simulink model "PowerTransmissionModel"  (R2024b)
settings: Solver=VariableStepAuto  StartTime=0.0  StopTime=1  RelTol=1e-3
libraries: fl_lib x17, ee_lib x10, nesl_utility x7
settings Model: Creator=pvenupra  LastModifiedBy=alial

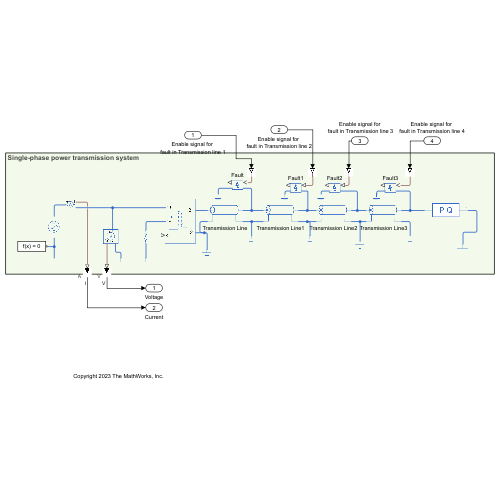
[thumbnail: Simulink's stored preview of the top-level diagram]
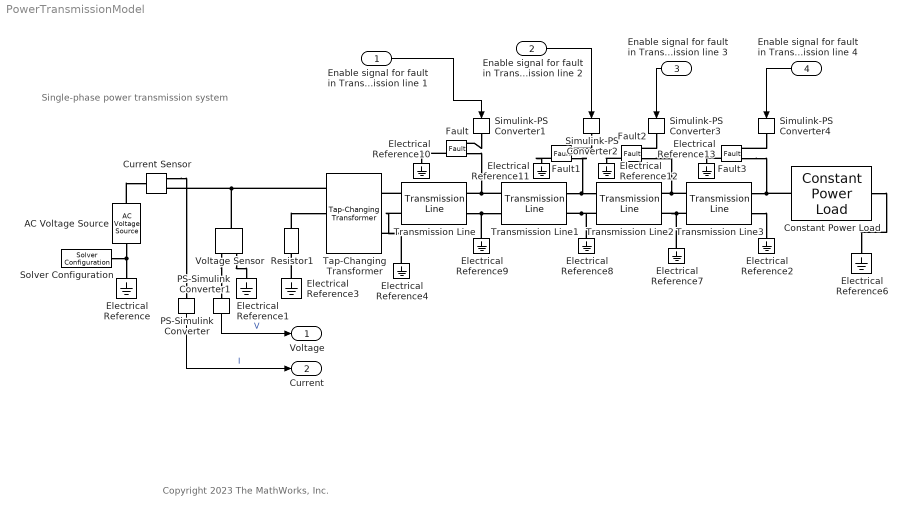
== system PowerTransmissionModel ==
  note: Copyright 2023 The MathWorks, Inc.
  note: Single-phase power transmission system
  Enable signal for fault in Transmission line 1 : Inport  SampleTime=0.025
  Enable signal for fault in Transmission line 2 : Inport  Port=2  SampleTime=0.025
  Enable signal for fault in Transmission line 3 : Inport  Port=3  SampleTime=0.025
  Enable signal for fault in Transmission line 4 : Inport  Port=4  SampleTime=0.025
  AC Voltage Source : fl_lib/Electrical/Electrical Sources/AC Voltage Source  amp=10 kV  shift=0 deg  frequency=60 Hz
  Constant Power Load : ee_lib/Passive/Constant Power Load  load_type=ee.enum.dc_ac.ac  consumed_power=100 W  min_supply_voltage=20 V  G_reverse=1e-6 S  deltaV=1e-3 V  active_power=4e5 W  reactive_power=1e5 A*V  f0=60 Hz  Vrms_min=400 V  tau=0.01 s  Vrms_ini=400 V  Vang_ini=0 deg  fault_action=simscape.enum.assert.action.none  t_fault=1 s
      settings: InternalSimscapePortConfiguration="{\"Bottom\":[],\"Left\":[{\"id\":\"p\",\"label\":\"+\",\"type\":\"foundation.electrical.electrical\"}],\"Right\":[{\"id\":\"n\",\"label\":\"-\",\"type\":\"foundation.electrical.electrical\"}],\"Top\":[]}"
  Current Sensor : fl_lib/Electrical/Electrical Sensors/Current Sensor
  Electrical Reference{,1..4,6..13} (13 alike) : fl_lib/Electrical/Electrical Elements/Electrical Reference
  Fault{,1..3} (4 alike) : ee_lib/Utilities/Fault  R_unfaulted=inf Ohm  R_faulted=1e-3 Ohm  fault_action=1  enable_temporal_fault=0  t_fault=0.3 s  fault_duration=inf s  enable_behavioral_fault=0  permissible_voltage_range=[-100, 100] V  t_fail_on_voltage=1 s  permissible_current_range=[-1, 1] A  t_fail_on_current=1 s  enable_external_fault=1  fault_condition=1  fault_threshold=0.5  fault_resettable=1
      settings: InternalSimscapePortConfiguration="{\"Bottom\":[],\"Left\":[{\"id\":\"p\",\"label\":\"+\",\"type\":\"foundation.electrical.electrical\"},{\"id\":\"F\",\"label\":\"F\",\"type\":\"input\"}],\"Right\":[{\"id\":\"n\",\"label\":\"-\",\"type\":\"foundation.electrical.electrical\"},{\"id\":\"X\",\"label\":\"X\",\"type\":\"output\"}],\"Top\":[]}"
  PS-Simulink Converter : nesl_utility/PS-Simulink Converter  PhysicalDomain=network_engine_domain  SubClassName=ps_output  LeftPortType=input  RightPortType=output  PseudoPeriodic=off  Frequencies=[]  VectorFormat=1-D array  Unit=A  AffineConversion=off
  PS-Simulink Converter1 : nesl_utility/PS-Simulink Converter  PhysicalDomain=network_engine_domain  SubClassName=ps_output  LeftPortType=input  RightPortType=output  PseudoPeriodic=off  Frequencies=[]  VectorFormat=1-D array  Unit=V  AffineConversion=off
  Resistor1 : fl_lib/Electrical/Electrical Elements/Resistor  R=0.2 Ohm  i_specify=off  i_priority=None  i=0 A  i_nominal_specify=off  i_nominal_value=1  i_nominal_unit=A  v_specify=off  v_priority=None  v=0 V  v_nominal_specify=off  v_nominal_value=1  v_nominal_unit=V
  Simulink-PS Converter{1..4} (4 alike) : nesl_utility/Simulink-PS Converter  PhysicalDomain=network_engine_domain  SubClassName=ps_input  LeftPortType=input  RightPortType=output  PseudoPeriodic=off  Frequencies=[]  NoiseDistribution=none  NoiseParameters=[]  Unit=1  AffineConversion=off  FilteringAndDerivatives=provide  SimscapeFilterOrder=1  InputFilterTimeConstant=0.001  UdotUserProvided=0
  Solver Configuration : nesl_utility/Solver Configuration  PhysicalDomain=network_engine_domain  SubClassName=solver  LeftPortType=input  RightPortType=generic  Tones=[]  Harmonics=[]  SimulateNoise=off  Profile=off  UseLocalSampling=off  EnableSwitchedLinearOptims=on  FrequencyDomain=off  UseCCode=off  RelTol=0.001  AbsTol=1e-06  MinStep=1e-09  ToWorkspace=off  RevertToSquareIcSolve=off  NumHomotopyIterations=100  PhasorMode=off  PhasorModeNumHarmonics=1  ConsistencySolver=NEWTON_FTOL  IndexReductionMethod=DerivativeReplacement  DoDC=off  ResidualTolerance=1e-09  ConsistencyTolSource=GLOBAL  ConsistencyAbsTol=0.001  ConsistencyRelTol=0.001  ConsistencyTolFactor=0.001  UseLocalSolver=on  LocalSolverChoice=NE_BACKWARD_EULER_ADVANCER  ResolveIndetEquations=on  FunctionEvalNumThread=1  LocalSolverSampleTime=1e-4  DoFixedCost=on  MaxNonlinIter=3  MaxModeIter=2  ComputeImpulses=off  ImpulseIterations=2  LinearAlgebra=auto  LinearAlgebraNumThread=0  EquationFormulation=NE_TIME_EF  DelaysMemoryBudget=1024  AutomaticFiltering=on  FilteringTimeConstant=0.001  PartitionStorageMethod=AS_NEEDED  PartitionMemoryBudget=1024  PartitionMethod=FAST  MultibodyUseLocalSolver=off  MultibodyLocalSolverChoice=ODE1  MultibodyLocalSolverSampleTime=0.001
  Tap-Changing Transformer : ee_lib/Passive/Transformers/Tap-Changing Transformer  n0=25  Lp=0.0133 H  Ls=2.12e-6 H  Rm=50 kOhm  Lm=132.63 H  Rp=2 Ohm  Rs="0.032  Ohm"  Gp=0 1/Ohm  Gs=0 1/Ohm  prm=1  pmin=-5  pmax=5  delta=1  controlThreshold=0.5  i1_specify=off  i1_priority=None  i1=0 A  i1_nominal_specify=off  i1_nominal_value=1  i1_nominal_unit=A  i2_specify=off  i2_priority=None  i2=0 A  i2_nominal_specify=off  i2_nominal_value=1  i2_nominal_unit=A  tapPosition_specify=off  tapPosition_priority=High  tapPosition=0
      settings: InternalSimscapePortConfiguration="{\"Bottom\":[],\"Left\":[{\"id\":\"p1\",\"label\":\"1+\",\"type\":\"foundation.electrical.electrical\"},{\"id\":\"n1\",\"label\":\"1-\",\"type\":\"foundation.electrical.electrical\"},{\"id\":\"control\",\"label\":\"c\",\"type\":\"input\"}],\"Right\":[{\"id\":\"p2\",\"label\":\"2+\",\"type\":\"foundation.electrical.electrical\"},{\"id\":\"n2\",\"label\":\"2-\",\"type\":\"foundation.electrical.electrical\"}],\"Top\":[]}"
  Transmission Line : ee_lib/Passive/Lines/Transmission Line  model_type=4  TD=5 ns  LC_param=2  Z0_delay_based=50 Ohm  Z0=50 Ohm  freq=60 Hz  Ll=220 uH/m  L=0.5 mH/km  C=0.3 uF/km  R=.2 Ohm/km  G=5e-6 S/m  LEN=0.1 km  N=1
      settings: InternalSimscapePortConfiguration="{\"Bottom\":[],\"Left\":[{\"id\":\"p1\",\"label\":\"\",\"type\":\"foundation.electrical.electrical\"},{\"id\":\"n1\",\"label\":\"\",\"type\":\"foundation.electrical.electrical\"}],\"Right\":[{\"id\":\"p2\",\"label\":\"\",\"type\":\"foundation.electrical.electrical\"},{\"id\":\"n2\",\"label\":\"\",\"type\":\"foundation.electrical.electrical\"}],\"Top\":[]}"
  Transmission Line1 : ee_lib/Passive/Lines/Transmission Line  model_type=4  TD=5 ns  LC_param=2  Z0_delay_based=50 Ohm  Z0=50 Ohm  freq=60 Hz  Ll=220 uH/m  L=0.5 mH/km  C=0.3 uF/km  R=.2 Ohm/km  G=5e-6 S/m  LEN=0.1 km  N=1
      settings: InternalSimscapePortConfiguration="{\"Bottom\":[],\"Left\":[{\"id\":\"p1\",\"label\":\"\",\"type\":\"foundation.electrical.electrical\"},{\"id\":\"n1\",\"label\":\"\",\"type\":\"foundation.electrical.electrical\"}],\"Right\":[{\"id\":\"p2\",\"label\":\"\",\"type\":\"foundation.electrical.electrical\"},{\"id\":\"n2\",\"label\":\"\",\"type\":\"foundation.electrical.electrical\"}],\"Top\":[]}"
  Transmission Line2 : ee_lib/Passive/Lines/Transmission Line  model_type=4  TD=5 ns  LC_param=2  Z0_delay_based=50 Ohm  Z0=50 Ohm  freq=60 Hz  Ll=220 uH/m  L=0.5 mH/km  C=0.3 uF/km  R=.2 Ohm/km  G=5e-6 S/m  LEN=0.1 km  N=1
      settings: InternalSimscapePortConfiguration="{\"Bottom\":[],\"Left\":[{\"id\":\"p1\",\"label\":\"\",\"type\":\"foundation.electrical.electrical\"},{\"id\":\"n1\",\"label\":\"\",\"type\":\"foundation.electrical.electrical\"}],\"Right\":[{\"id\":\"p2\",\"label\":\"\",\"type\":\"foundation.electrical.electrical\"},{\"id\":\"n2\",\"label\":\"\",\"type\":\"foundation.electrical.electrical\"}],\"Top\":[]}"
  Transmission Line3 : ee_lib/Passive/Lines/Transmission Line  model_type=4  TD=5 ns  LC_param=2  Z0_delay_based=50 Ohm  Z0=50 Ohm  freq=60 Hz  Ll=220 uH/m  L=0.1 mH/km  C=0.3 uF/km  R=.02 Ohm/km  G=5e-6 S/m  LEN=0.1 km  N=1
      settings: InternalSimscapePortConfiguration="{\"Bottom\":[],\"Left\":[{\"id\":\"p1\",\"label\":\"\",\"type\":\"foundation.electrical.electrical\"},{\"id\":\"n1\",\"label\":\"\",\"type\":\"foundation.electrical.electrical\"}],\"Right\":[{\"id\":\"p2\",\"label\":\"\",\"type\":\"foundation.electrical.electrical\"},{\"id\":\"n2\",\"label\":\"\",\"type\":\"foundation.electrical.electrical\"}],\"Top\":[]}"
  Voltage Sensor : fl_lib/Electrical/Electrical Sensors/Voltage Sensor
  Voltage : Outport
  Current : Outport  Port=2
  wires:
  PS-Simulink Converter1/1 -> Voltage/1  "V"
  PS-Simulink Converter/1 -> Current/1  "I"
  Enable signal for fault in Transmission line 2/1 -> Simulink-PS Converter2/1
  Enable signal for fault in Transmission line 3/1 -> Simulink-PS Converter3/1
  Enable signal for fault in Transmission line 4/1 -> Simulink-PS Converter4/1
  Enable signal for fault in Transmission line 1/1 -> Simulink-PS Converter1/1
  connections:
  AC Voltage Source/RConn1 -- Electrical Reference/LConn1 -- Solver Configuration/RConn1
  Electrical Reference4/LConn1 -- Transmission Line/LConn2 -- Tap-Changing Transformer/RConn2
  Transmission Line/LConn1 -- Tap-Changing Transformer/RConn1
  Current Sensor/RConn1 -- PS-Simulink Converter/LConn1
  Tap-Changing Transformer/LConn1 -- Voltage Sensor/LConn1 -- Current Sensor/RConn2
  Voltage Sensor/RConn1 -- PS-Simulink Converter1/LConn1
  Voltage Sensor/RConn2 -- Electrical Reference1/LConn1
  AC Voltage Source/LConn1 -- Current Sensor/LConn1
  Resistor1/RConn1 -- Tap-Changing Transformer/LConn2
  Electrical Reference3/LConn1 -- Resistor1/LConn1
  Transmission Line2/LConn2 -- Electrical Reference8/LConn1 -- Transmission Line1/RConn2
  Transmission Line3/LConn1 -- Fault2/LConn1 -- Transmission Line2/RConn1
  Transmission Line3/LConn2 -- Electrical Reference7/LConn1 -- Transmission Line2/RConn2
  Transmission Line/RConn2 -- Transmission Line1/LConn2 -- Electrical Reference9/LConn1
  Transmission Line3/RConn2 -- Electrical Reference2/LConn1
  Transmission Line1/LConn1 -- Fault/LConn1 -- Transmission Line/RConn1
  Transmission Line1/RConn1 -- Fault1/LConn1 -- Transmission Line2/LConn1
  Transmission Line3/RConn1 -- Fault3/LConn1 -- Constant Power Load/LConn1
  Constant Power Load/RConn1 -- Electrical Reference6/LConn1
  Fault/RConn1 -- Electrical Reference10/LConn1
  Simulink-PS Converter1/RConn1 -- Fault/LConn2
  Fault1/RConn1 -- Electrical Reference11/LConn1
  Simulink-PS Converter2/RConn1 -- Fault1/LConn2
  Fault2/RConn1 -- Electrical Reference12/LConn1
  Simulink-PS Converter3/RConn1 -- Fault2/LConn2
  Fault3/RConn1 -- Electrical Reference13/LConn1
  Simulink-PS Converter4/RConn1 -- Fault3/LConn2
